simulink model "Gegen_und_Mitkopplung"  (Simulink 8.3)
settings: Solver=ode23  SolverMode=SingleTasking  StartTime=0  StopTime=20  MaxStep=0.1  RelTol=1e-3  AbsTol=1e-6
PreLoadFcn:
  | zeta=0.2;wn=1;
libraries: simulink x1, cstblocks x1
settings Model: Creator=bruhm  LastModifiedBy=Bruhm  ExtModeTrigMode=oneshot  ExtModeArmWhenConnect=off
settings DataIOCC: ExternalInput=[]  InitialState=[]  LimitDataPoints=off  SaveOutput=off  SaveTime=off  SignalLoggingName=sigsOut
settings OptimizationCC: BooleanDataType=off  ExpressionDepthLimit=2147483647  InitFltsAndDblsToZero=on
settings DebuggingCC: SaveWithParameterizedLinksMsg=none  SignalResolutionControl=TryResolveAllWithWarning  SolverPrmCheckMsg=none  MultiTaskDSMMsg=warning  MultiTaskCondExecSysMsg=none  FcnCallInpInsideContextMsg=UseLocalSettings
settings HardwareCC: TargetUnknown=on
settings RTWCC: IncludeERTFirstTime=on
settings GRTTargetCC: TargetFcnLib=ansi_tfl_tmw.mat

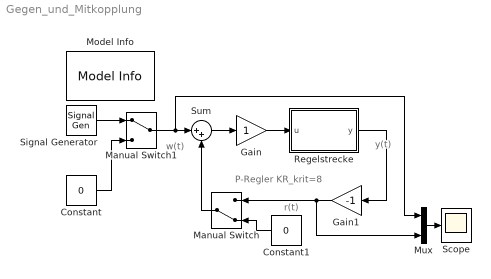
== system Gegen_und_Mitkopplung ==
  note: w(t)
  note: P-Regler
      | KR_krit=8
  note: y(t)
  note: r(t)
  Constant : Constant  Value=0
  Constant1 : Constant  Value=0
  Gain : Gain  SaturateOnIntegerOverflow=on  OutDataTypeStr=Inherit: Same as input  ParamDataTypeStr=Inherit: Same as input
  Gain1 : Gain  Gain=-1  SaturateOnIntegerOverflow=on  OutDataTypeStr=Inherit: Same as input  ParamDataTypeStr=Inherit: Same as input
  Manual Switch : ManualSwitch  CurrentSetting=0
  Manual Switch1 : ManualSwitch
  Model Info : simulink/Model-Wide Utilities/Model Info  InitialBlockCM=None  BlockCM=none  Frame=off  DisplayStringWithTags=|  HorizontalTextAlignment=Left  LeftAlignmentValue=0.02  SourceBlockDiagram=Gegen_und_Mitkopplung  TagMaxNumber=20
      | f1 = 0.1 Hz
      | f2 = 0.2 Hz
      | f3 = 0.4 Hz
      | f4 = f_krit = 0.5513 Hz
  Mux : Mux  Inputs=3
  Regelstrecke : Subsystem
  Scope : Scope
      settings: TimeRange=20  YMin=-2  YMax=2
  Signal Generator : SignalGenerator  Frequency=0.1
  Sum : Sum  Inputs=|++  SaturateOnIntegerOverflow=on  InputSameDT=on  OutDataTypeStr=Inherit: Same as first input
  wires:
  Signal Generator/1 -> Manual Switch1/1
  Sum/1 -> Gain/1
  Manual Switch/1 -> Sum/2
  Gain/1 -> Regelstrecke/1(u)
  Gain1/1 -> Manual Switch/1, Mux/3
  Regelstrecke/1(y) -> Gain1/1
  Constant/1 -> Manual Switch1/2
  Constant1/1 -> Manual Switch/2
  Mux/1 -> Scope/1
  Manual Switch1/1 -> Mux/1, Sum/1

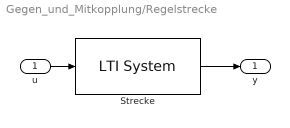
== system Gegen_und_Mitkopplung/Regelstrecke ==
  u : Inport
  Strecke : cstblocks/LTI System  sys=ss(zpk([],[-2 -2 -2],8))  IC=[-0.5 0 0]
  y : Outport
  wires:
  Strecke/1 -> y/1
  u/1 -> Strecke/1
